simulink model "Lorentza"  (R2023b)
settings: Solver=VariableStepAuto  StartTime=0.0  StopTime=10.0  RelTol=1e-3
settings Model: Creator=golde  LastModifiedBy=golde

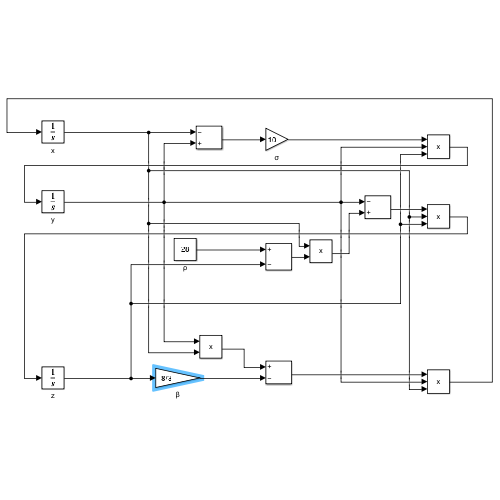
[thumbnail: Simulink's stored preview of the top-level diagram]
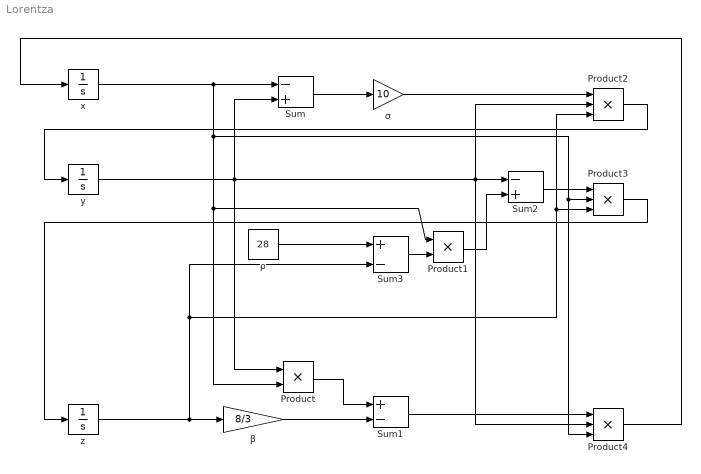
== system Lorentza ==
  Product : Product
  Product1 : Product
  Product2 : Product  Inputs=3
  Product3 : Product  Inputs=3
  Product4 : Product  Inputs=3
  Sum : Sum  Inputs=-+
  Sum1 : Sum  Inputs=+-
  Sum2 : Sum  Inputs=-+
  Sum3 : Sum  Inputs=+-
  x : Integrator  InitialCondition=1
  y : Integrator  InitialCondition=1
  z : Integrator  InitialCondition=1
  β : Gain  Gain=8/3
  ρ : Constant  Value=28
  σ : Gain  Gain=10
  wires:
  x/1 -> Product1/1, Product/2, Product3/2, Product4/3, Sum/1
  y/1 -> Product2/2, Product4/2, Sum2/1, Product/1, Sum/2
  Sum/1 -> σ/1
  z/1 -> Product2/3, Product3/3, Sum3/2, β/1
  β/1 -> Sum1/2
  Product/1 -> Sum1/1
  ρ/1 -> Sum3/1
  Sum3/1 -> Product1/2
  Product1/1 -> Sum2/2
  σ/1 -> Product2/1
  Sum2/1 -> Product3/1
  Sum1/1 -> Product4/1
  Product2/1 -> y/1
  Product3/1 -> z/1
  Product4/1 -> x/1
